simulink model "R0005E_Cascade"  (R2020a)
settings: Solver=ode5  StartTime=0.0  StopTime=inf  RelTol=1e-3  EnableMultiTasking=on
undefined symbols (not defined in the file): DiscIntNeverNeededParam, National_Instruments, PCI
libraries: sldrtlib x2, simulink x2
settings Model: Creator=wolfgang  LastModifiedBy=Wolfgang
settings Model: ModifiedHistory=|
  | Created an adjusted empty Simulink diagram for the lab assignments
  | in the course R0002E
settings DataIOCC: SaveFormat=Array  SignalLoggingSaveFormat=ModelDataLogs  SaveOutput=off  SignalLogging=off  DSMLogging=off  SaveTime=off  ReturnWorkspaceOutputs=off
settings OptimizationCC: ExpressionDepthLimit=2147483647  LifeSpan=inf
settings DebuggingCC: UnderspecifiedInitializationDetection=Classic  MergeDetectMultiDrivingBlocksExec=none  SolverPrmCheckMsg=warning  FcnCallInpInsideContextMsg=warning  StateNameClashWarn=warning  SFUnexpectedBacktrackingDiag=warning  SFNoUnconditionalDefaultTransitionDiag=warning  SFExecutionAtInitializationDiag=none  ArithmeticOperatorsInVariantConditions=warning
settings HardwareCC: ProdBitPerPointer=32  ProdBitPerSizeT=32  ProdBitPerPtrDiffT=32  ProdLargestAtomicFloat=None  ProdIntDivRoundTo=Undefined  ProdEndianess=Unspecified  ProdWordSize=32  ProdHWDeviceType=32-bit Generic
settings ModelReferenceCC: PropagateSignalLabelsOutOfModel=off
settings SFSimCC: SimUseLocalCustomCode=off  CustomCodeUndefinedFunction=UseInterfaceOnly
settings RTWCC: RTWUseLocalCustomCode=off
settings CodeAppCC: StateflowObjectComments=on
settings GRTTargetCC: TargetLangStandard=C89/C90 (ANSI)
settings ConfigComp: CovMetricSettings=dw  CovHtmlReporting=on  CovSaveCumulativeToWorkspaceVar=on  CovSaveSingleToWorkspaceVar=on  CovExternalEMLEnable=off  CovSFcnEnable=off

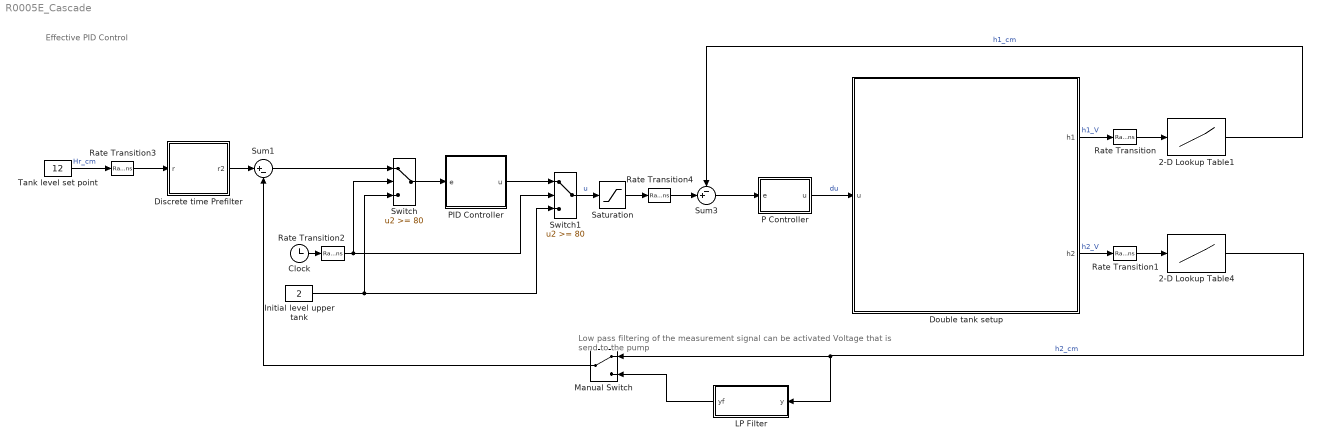
== system R0005E_Cascade ==
  note: Effective PID Control
  note: Low pass filtering of the measurement signal can be activated
      |
      |
      |
      |
      | Voltage that is send to the pump
  2-D Lookup Table1 : Lookup_n-D  NumberOfTableDimensions=1  BreakpointsForDimension1=x  BreakpointsForDimension2=[1:3]  Table=y  RndMeth=Simplest  InputSameDT=on  mask{x=[0.21,0.62,1.00,1.49,1.80,2.12,2.54,2.97,3.32,3.71,4.09,4.51,4.87,5.25,5.57,6.04,6.41,6.78,7.13,7.56,7.91,8.32,8.69,9.07,9.42,9.82,9.99], y=[2.50,3.00,3.50,4.00,4.50,5.00,5.50,6.00,6.50,7.00,7.50,8.00,8.50,9.00,9.50,10.00,10.50,11.00,11.50,12.00,12.50,13.00,13.50,14.00,14.50,15.00,15.50]}
      mask prompts: x "Values on x-axis"; y "Values on y-axis"
  2-D Lookup Table4 : Lookup_n-D  NumberOfTableDimensions=1  BreakpointsForDimension1=x  BreakpointsForDimension2=[1:3]  Table=y  RndMeth=Simplest  InputSameDT=on  mask{x=[0.21,0.62,1.00,1.49,1.80,2.12,2.54,2.97,3.32,3.71,4.09,4.51,4.87,5.25,5.57,6.04,6.41,6.78,7.13,7.56,7.91,8.32,8.69,9.07,9.42,9.82,9.99], y=[2.50,3.00,3.50,4.00,4.50,5.00,5.50,6.00,6.50,7.00,7.50,8.00,8.50,9.00,9.50,10.00,10.50,11.00,11.50,12.00,12.50,13.00,13.50,14.00,14.50,15.00,15.50]}
      mask prompts: x "Values on x-axis"; y "Values on y-axis"
  Clock : Clock
  Discrete time Prefilter : Subsystem  mask(Discrete time prefilter){beta=3, alpha0=0.1, alpha1=30, alpha2=2, Ts=0.5}
      mask prompts: beta "beta (numerator gain)"; Ts "Sample time [s]"
      mask help: Discrete time realization of a pre-filter with no zeros and of second order. Intended to compensate for the zeros of a closed loop system with two left half plane zeros
  Double tank setup : Subsystem  AncestorBlock=R0002E_lib/Double tank setup  StopFcn=|  mask(Realtime interface for the tank process){ts=0.02, h1_ch=0, h2_ch=1, u_ch=0}
      | chn =get_param(gcb,'u_ch');                          
      | s = daq.createSession('ni');                         
      | channel = ['ao',chn];                                
      | s.addAnalogOutputChannel('Dev1', channel, 'Voltage');
      | x = zeros(5,1);                                      
      | s.queueOutputData(x);                                
      | lh = s.addlistener('DataRequired', ...               
      | @(src,event) src.queueOutputData(x));                
      | s.startBackground();                                 
      | s.wait();                                            
      | s.stop();                                            
      | delete(lh);                                          
      | clear chn;                                           
      | clear s;                                             
      | clear channel;                                       
      | clear lh;                                            
      | clear x;
      mask prompts: ts "Sample time"; h1_ch "A/D Channel for upper tank"; h2_ch "A/D Channel for lower tank"; u_ch "D/A Channel for pump"
      mask help:
      | This block represents the physical interface from the computer to the tank process.
      |
      | The input u is the voltage that is provided for the pump, the output h1 is the measured level in the upper tank in [V] and the output h2 is the
      | measured level in the lower tank in [V].
      |
      | You need to provide the sample rate at which the voltage to the pump is updated and the level measurements are sampled. The sample rate should not be less than 0.02 seconds.
      mask Display:
      | x=363;
      | y=381;
      | image(imread('tank_icon.jpg'));
      | text(250/x,309/y,'Sensor');
      | text(260/x,169/y,'Sensor');
      | text(335/x,289/y,'A');
      | text(351/x,283/y,'D');
      | text(335/x,100/y,'A');
      | text(351/x,95/y,'D');
      | text(22/x,187/y,'A');
      | text(5/x,195/y,'D');
      | text(225/x,278/y,'h_1','texmode','on');
      | text(225/x,146/y,'h_2','texmode','on');
      | text(300/x,270/y,sprintf('AI-%d',h1_ch));
      | text(300/x,80/y,sprintf('AI-%d',h2_ch));
      | text(40/x,173/y,sprintf('AO-%d',u_ch));
  Initial level upper tank : Constant  Value=2  SampleTime=0.5
  LP Filter : Subsystem  mask{Tf=1, Ts=0.02}
      mask prompts: Tf "Time constant"; Ts "Sampling time"
      mask help: First order low pass filter.
      mask Display: disp('LP')
  Manual Switch : ManualSwitch
  P Controller : Subsystem  mask(Simple PID Controller){kP=3, kI=0, kD=0, u0=2, Ts=0.1}
      mask prompts: kP "Proportional Gain kP"; kI "Integral Gain kI"; kD "Derivative Gain kD"; u0 "Operating point pump speed"; Ts "Sample time [s]"
      mask help:
      | Parameter setting for a PID controller in parallel implementation with
      | the parameters kP, kI and kD. The controller also makes use of the operating
      | point for the pump speed, called u0.
  PID Controller : Subsystem  mask(Simple PID Controller){kP=3, kI=0.1, kD=30, u0=2, Ts=0.5}
      mask prompts: kP "Proportional Gain kP"; kI "Integral Gain kI"; kD "Derivative Gain kD"; u0 "Operating point pump speed"; Ts "Sample time [s]"
      mask help:
      | Parameter setting for a PID controller in parallel implementation with
      | the parameters kP, kI and kD. The controller also makes use of the operating
      | point for the pump speed, called u0.
  Rate Transition : RateTransition  OutPortSampleTime=0.1
  Rate Transition1 : RateTransition  OutPortSampleTime=0.5
  Rate Transition2 : RateTransition  OutPortSampleTime=0.5
  Rate Transition3 : RateTransition  OutPortSampleTime=0.5
  Rate Transition4 : RateTransition  OutPortSampleTime=0.1
  Saturation : Saturate  UpperLimit=15  LowerLimit=0
  Sum1 : Sum  Inputs=|+-
  Sum3 : Sum  Inputs=-+|
  Switch : Switch  Threshold=80
  Switch1 : Switch  Threshold=80
  Tank level set point : Constant  Value=12  SampleTime=0.5
  wires:
  Tank level set point/1 -> Rate Transition3/1  "Hr_cm"
  2-D Lookup Table4/1 -> LP Filter/1(y), Manual Switch/1  "h2_cm"
  Double tank setup/2(h2) -> Rate Transition1/1  "h2_V"
  Double tank setup/1(h1) -> Rate Transition/1  "h1_V"
  2-D Lookup Table1/1 -> Sum3/1  "h1_cm"
  Switch/1 -> PID Controller/1(e)
  Clock/1 -> Rate Transition2/1
  PID Controller/1(u) -> Switch1/1
  Switch1/1 -> Saturation/1  "u"
  Sum1/1 -> Switch/1
  Initial level upper tank/1 -> Switch1/3, Switch/3
  Rate Transition/1 -> 2-D Lookup Table1/1
  Rate Transition1/1 -> 2-D Lookup Table4/1
  Rate Transition2/1 -> Switch1/2, Switch/2
  P Controller/1(u) -> Double tank setup/1(u)  "du"
  Sum3/1 -> P Controller/1(e)
  Saturation/1 -> Rate Transition4/1
  Discrete time Prefilter/1(r2) -> Sum1/1
  Rate Transition3/1 -> Discrete time Prefilter/1(r)
  Rate Transition4/1 -> Sum3/2
  Manual Switch/1 -> Sum1/2
  LP Filter/1(yf) -> Manual Switch/2

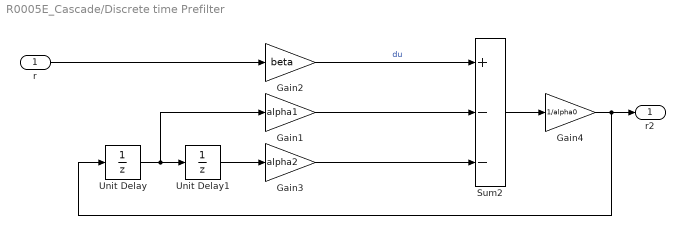
== system R0005E_Cascade/Discrete time Prefilter ==
  r : Inport
  Gain1 : Gain  Gain=alpha1
  Gain2 : Gain  Gain=beta
  Gain3 : Gain  Gain=alpha2
  Gain4 : Gain  Gain=1/alpha0
  Sum2 : Sum  Inputs=+--
  Unit Delay : UnitDelay  SampleTime=Ts  HasFrameUpgradeWarning=on
  Unit Delay1 : UnitDelay  SampleTime=Ts  HasFrameUpgradeWarning=on
  r2 : Outport
  wires:
  Gain3/1 -> Sum2/3
  Gain1/1 -> Sum2/2
  Unit Delay1/1 -> Gain3/1
  Unit Delay/1 -> Gain1/1, Unit Delay1/1
  r/1 -> Gain2/1
  Gain2/1 -> Sum2/1  "du"
  Sum2/1 -> Gain4/1
  Gain4/1 -> Unit Delay/1, r2/1

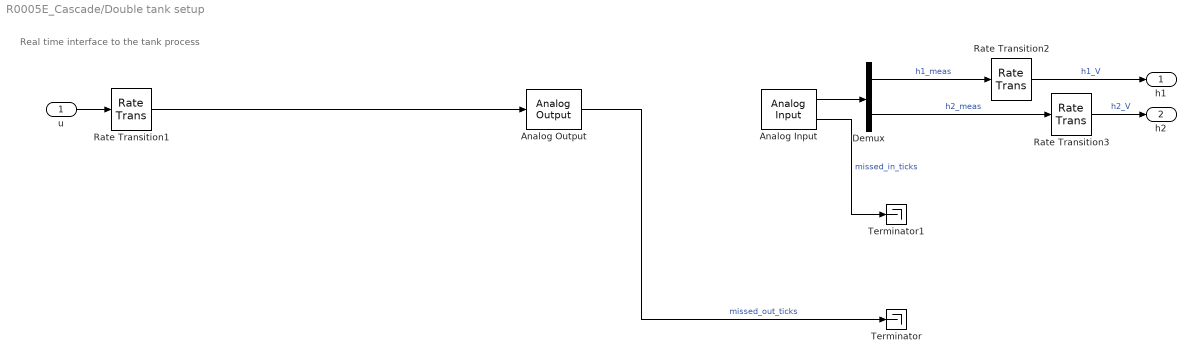
== system R0005E_Cascade/Double tank setup ==
  note: Real time interface to the tank process
  u : Inport
  Analog Input : sldrtlib/Analog Input  SampleTime=ts  MaxMissedTicks=500000000  ShowMissedTicks=on  YieldWhenWaiting=off  DrvName=National_Instruments/PCI-6024E  DrvAddress=4294967295  DrvOptions=[0 0 0 0 0 0]  Channels=[h1_ch+1,h2_ch+1]  RangeMode=1  VoltRange=1  DataType=1
      settings: AttributesFormatString=National Instruments\nPCI-6024E [auto]
  Analog Output : sldrtlib/Analog Output  SampleTime=ts  MaxMissedTicks=500000000  ShowMissedTicks=on  YieldWhenWaiting=off  DrvName=National_Instruments/PCI-6024E  DrvAddress=4294967295  DrvOptions=[0 0 0 0 0 0]  Channels=u_ch+1  RangeMode=1  VoltRange=1  InitialValue=0  FinalValue=0
      settings: AttributesFormatString=National Instruments\nPCI-6024E [auto]
  Demux : Demux  Outputs=2
  Rate Transition1 : RateTransition  OutPortSampleTime=ts
  Rate Transition2 : RateTransition
  Rate Transition3 : RateTransition
  Terminator : Terminator
  Terminator1 : Terminator
  h1 : Outport
  h2 : Outport  Port=2
  wires:
  Rate Transition1/1 -> Analog Output/1
  Rate Transition3/1 -> h2/1  "h2_V"
  Rate Transition2/1 -> h1/1  "h1_V"
  Analog Input/2 -> Terminator1/1  "missed_in_ticks"
  Demux/2 -> Rate Transition3/1  "h2_meas"
  Demux/1 -> Rate Transition2/1  "h1_meas"
  Analog Input/1 -> Demux/1
  Analog Output/1 -> Terminator/1  "missed_out_ticks"
  u/1 -> Rate Transition1/1

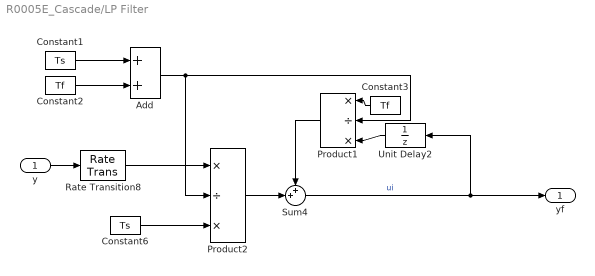
== system R0005E_Cascade/LP Filter ==
  y : Inport
  Add : Sum
  Constant1 : Constant  Value=Ts
  Constant2 : Constant  Value=Tf
  Constant3 : Constant  Value=Tf
  Constant6 : Constant  Value=Ts
  Product1 : Product  Inputs=*/*  RndMeth=Zero
  Product2 : Product  Inputs=*/*  RndMeth=Zero
  Rate Transition8 : RateTransition  OutPortSampleTime=Ts
  Sum4 : Sum  Inputs=++|
  Unit Delay2 : UnitDelay  SampleTime=-1  HasFrameUpgradeWarning=on
  yf : Outport
  wires:
  Sum4/1 -> Unit Delay2/1, yf/1  "ui"
  Product2/1 -> Sum4/2
  Product1/1 -> Sum4/1
  Unit Delay2/1 -> Product1/3
  y/1 -> Rate Transition8/1
  Constant6/1 -> Product2/3
  Rate Transition8/1 -> Product2/1
  Constant1/1 -> Add/1
  Constant2/1 -> Add/2
  Add/1 -> Product1/2, Product2/2
  Constant3/1 -> Product1/1

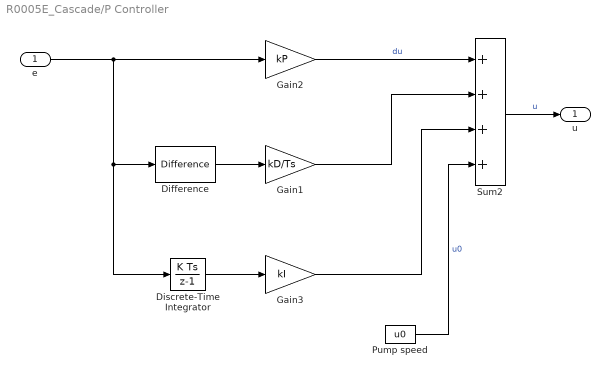
== system R0005E_Cascade/P Controller ==
  e : Inport
  Difference : simulink/Discrete/Difference  ICPrevInput=0.0  OutMin=[]  OutMax=[]  OutDataType=fixdt(1, 16)  OutScaling=2^-10  DoSatur=off
  Discrete-Time Integrator : DiscreteIntegrator  SampleTime=Ts  ICPrevOutput=DiscIntNeverNeededParam  ICPrevScaledInput=DiscIntNeverNeededParam
  Gain1 : Gain  Gain=kD/Ts
  Gain2 : Gain  Gain=kP
  Gain3 : Gain  Gain=kI
  Pump speed : Constant  Value=u0  SampleTime=Ts
  Sum2 : Sum  Inputs=++++
  u : Outport
  wires:
  Pump speed/1 -> Sum2/4  "u0"
  Gain3/1 -> Sum2/3
  Gain1/1 -> Sum2/2
  Discrete-Time Integrator/1 -> Gain3/1
  Difference/1 -> Gain1/1
  e/1 -> Gain2/1, Difference/1, Discrete-Time Integrator/1
  Gain2/1 -> Sum2/1  "du"
  Sum2/1 -> u/1  "u"

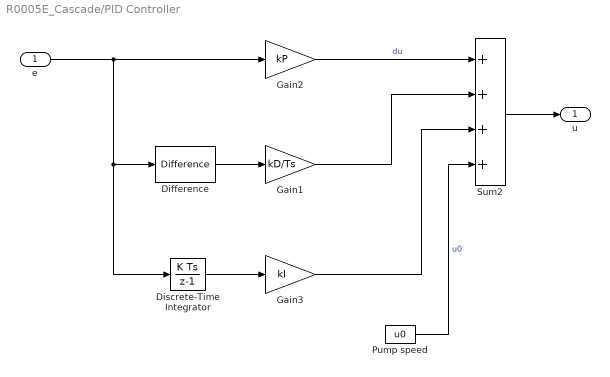
== system R0005E_Cascade/PID Controller ==
  e : Inport
  Difference : simulink/Discrete/Difference  ICPrevInput=0.0  OutMin=[]  OutMax=[]  OutDataType=fixdt(1, 16)  OutScaling=2^-10  DoSatur=off
  Discrete-Time Integrator : DiscreteIntegrator  SampleTime=Ts  ICPrevOutput=DiscIntNeverNeededParam  ICPrevScaledInput=DiscIntNeverNeededParam
  Gain1 : Gain  Gain=kD/Ts
  Gain2 : Gain  Gain=kP
  Gain3 : Gain  Gain=kI
  Pump speed : Constant  Value=u0  SampleTime=Ts
  Sum2 : Sum  Inputs=++++
  u : Outport
  wires:
  Sum2/1 -> u/1
  Gain2/1 -> Sum2/1  "du"
  e/1 -> Discrete-Time Integrator/1, Difference/1, Gain2/1
  Difference/1 -> Gain1/1
  Discrete-Time Integrator/1 -> Gain3/1
  Gain1/1 -> Sum2/2
  Gain3/1 -> Sum2/3
  Pump speed/1 -> Sum2/4  "u0"
